simulink model "cw7_model_Relidzynski"  (R2022a)
settings: Solver=VariableStepAuto  StartTime=1  StopTime=200  RelTol=1e-3
values from neighbouring files (symbols this model uses):
  a11 = -1/(R1*C1)    (= -0.1)    [cw7_dane_Relidzynski.m]
  a12 = 1/(R1*C1)    (= 0.1)    [cw7_dane_Relidzynski.m]
  a21 = 1/(R1*C2)    (= 0.2)    [cw7_dane_Relidzynski.m]
  a22 = -1/(R1*C2)-1/(R2*C2)    (= -0.4)    [cw7_dane_Relidzynski.m]
  b1 = 1/C1    (= 0.1)    [cw7_dane_Relidzynski.m]
settings Model: Creator=Radek  LastModifiedBy=Radosław

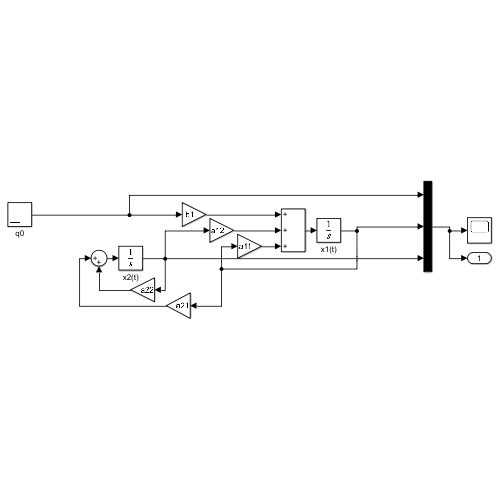
[thumbnail: Simulink's stored preview of the top-level diagram]
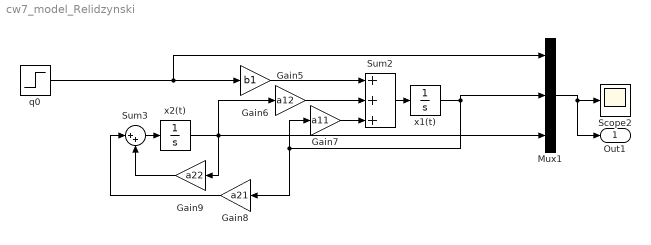
== system cw7_model_Relidzynski ==
  Gain5 : Gain  Gain=a12
  Gain6 : Gain  Gain=b1
  Gain7 : Gain  Gain=a11
  Gain8 : Gain  Gain=a21
  Gain9 : Gain  Gain=a22
  Mux1 : Mux  Inputs=3
  Scope2 : Scope
  Sum2 : Sum  Inputs=+++
  Sum3 : Sum  Inputs=|++
  q0 : Step  SampleTime=0
  x1(t) : Integrator
  x2(t) : Integrator
  Out1 : Outport
  wires:
  Gain7/1 -> Sum2/3
  Gain5/1 -> Sum2/2
  Sum3/1 -> x2(t)/1
  Sum2/1 -> x1(t)/1
  x1(t)/1 -> Gain8/1, Gain7/1, Mux1/2
  q0/1 -> Mux1/1, Gain6/1
  x2(t)/1 -> Mux1/3, Gain5/1, Gain9/1
  Gain8/1 -> Sum3/1
  Mux1/1 -> Out1/1, Scope2/1
  Gain9/1 -> Sum3/2
  Gain6/1 -> Sum2/1
